simulink model "Backsteping2_Tanques_2_Des"  (R2025b)
settings: Solver=VariableStepAuto  StartTime=0.0  StopTime=10.0  RelTol=1e-3
settings Model: Creator=Sthev  LastModifiedBy=ACER

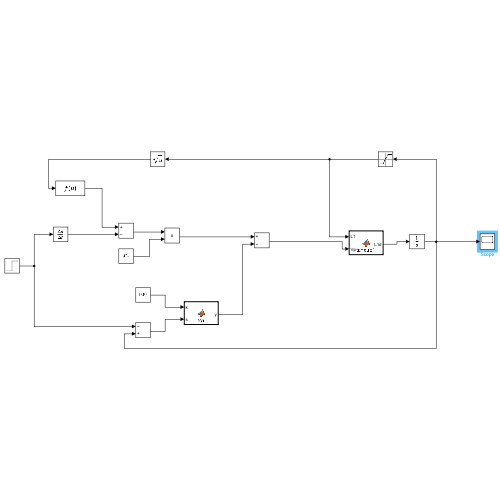
[thumbnail: Simulink's stored preview of the top-level diagram]
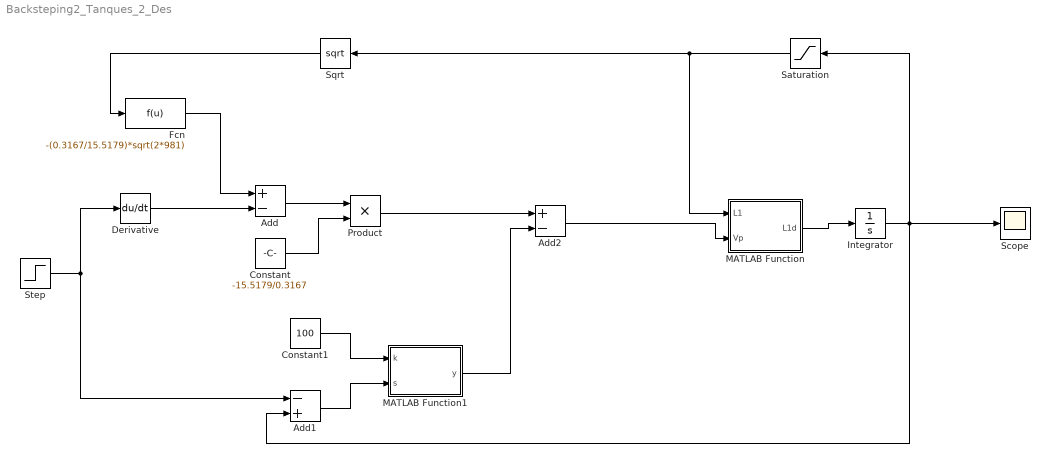
== system Backsteping2_Tanques_2_Des ==
  Add : Sum  Inputs=+-
  Add1 : Sum  Inputs=-+
  Add2 : Sum  Inputs=+-
  Constant : Constant  Value=-15.5179/0.3167
  Constant1 : Constant  Value=100
  Derivative : Derivative
  Fcn : Fcn  Expr=-(0.3167/15.5179)*sqrt(2*981)
  Integrator : Integrator
  MATLAB Function : MATLAB Function  TreatAsAtomicUnit=on
  MATLAB Function1 : MATLAB Function  TreatAsAtomicUnit=on
  Product : Product
  Saturation : Saturate  UpperLimit=24  LowerLimit=0
  Scope : Scope
      settings: ActiveDisplayYMinimum=-1.8960654199527522  ActiveDisplayYMaximum=17.064588779574773
  Sqrt : Sqrt
  Step : Step  Time=0  After=15  SampleTime=0
  wires:
  Derivative/1 -> Add/2
  Fcn/1 -> Add/1
  Sqrt/1 -> Fcn/1
  Saturation/1 -> MATLAB Function/1(L1), Sqrt/1
  MATLAB Function/1(L1d) -> Integrator/1
  Integrator/1 -> Scope/1, Add1/2, Saturation/1
  Constant/1 -> Product/2
  Add/1 -> Product/1
  Step/1 -> Derivative/1, Add1/1
  Constant1/1 -> MATLAB Function1/1(k)
  Add1/1 -> MATLAB Function1/2(s)
  MATLAB Function1/1(y) -> Add2/2
  Product/1 -> Add2/1
  Add2/1 -> MATLAB Function/2(Vp)

== matlab function Backsteping2_Tanques_2_Des/MATLAB Function ==
  data: L1 input; L1d output; Vp input
% Sistema tanque
function L1d =tanque1(L1,Vp)
% xd=f(x,u)
% tanque1(u(1),u(02))

% Parametros
dt1=4.445; %cm
d01=0.635; %cm
At1=pi*dt1^2/4;  % ajustar
A01=pi*d01^2/4;
kp = 3.3;
g=980;  % cm/s2

% flujo de salida
v01=sqrt(2*g*L1);   % velocidad de flujo de salida
F01=A01*v01;          % flujo de salida
Fi1=kp*Vp;          % flujo de entrada

% modelo no lineal A*dL1/dt=Fi1 - F01
L1d=Fi1/At1-F01/At1;

== matlab function Backsteping2_Tanques_2_Des/MATLAB Function1 ==
  data: k input; y output; s input
function y = fcn(k, s)
r=0;
if s>0
    r = k;
end
if s<0
    r = -k;
end
y = r;
